simulink model "dlbsTestHarnessMatrixMultiply"  (R2025b)
settings: Solver=VariableStepAuto  StartTime=0.0  StopTime=10.0  RelTol=1e-3
undefined symbols (not defined in the file or in its folder): dY, W, X
libraries: dlbsBlockExtractGradientGF x2, dlbsBlockInsertGradientGF x1, dlbsBlockMatrixMultiply x1
settings Model: Creator=lt6037  LastModifiedBy=lt6037

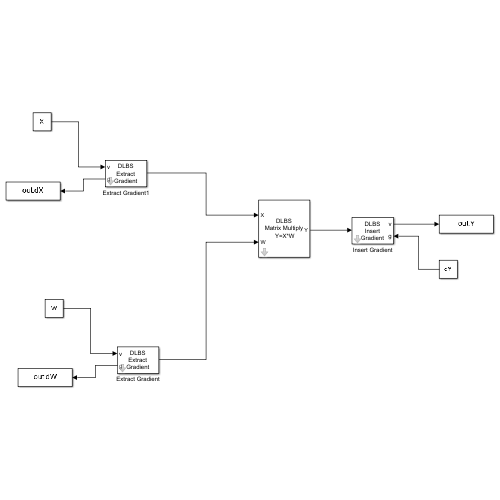
[thumbnail: Simulink's stored preview of the top-level diagram]
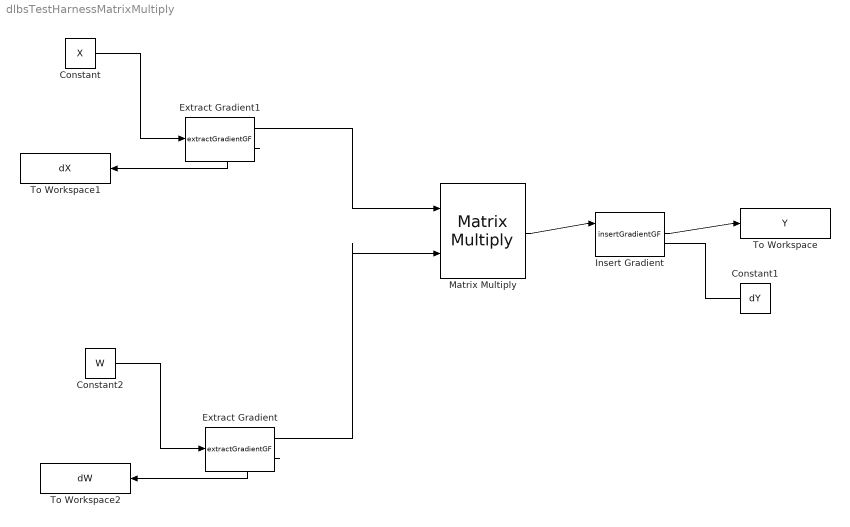
== system dlbsTestHarnessMatrixMultiply ==
  Constant : Constant  Value=X  VectorParams1D=off
  Constant1 : Constant  Value=dY  VectorParams1D=off
  Constant2 : Constant  Value=W  VectorParams1D=off
  Extract Gradient : dlbsBlockExtractGradientGF/extractGradientGF
  Extract Gradient1 : dlbsBlockExtractGradientGF/extractGradientGF
  Insert Gradient : dlbsBlockInsertGradientGF/insertGradientGF
  Matrix Multiply : dlbsBlockMatrixMultiply/Matrix Multiply
  To Workspace : ToWorkspace  VariableName=Y  SaveFormat=Timeseries  SampleTime=-1
      settings: MaxDataPoints=1
  To Workspace1 : ToWorkspace  VariableName=dX  SaveFormat=Timeseries  SampleTime=-1
      settings: MaxDataPoints=1
  To Workspace2 : ToWorkspace  VariableName=dW  SaveFormat=Timeseries  SampleTime=-1
      settings: MaxDataPoints=1
  wires:
  Extract Gradient1/2 -> To Workspace1/1
  Constant1/1 -> Insert Gradient/2
  Constant/1 -> Extract Gradient1/1
  Insert Gradient/1 -> To Workspace/1
  Extract Gradient/2 -> To Workspace2/1
  Constant2/1 -> Extract Gradient/1
  Extract Gradient1/1 -> Matrix Multiply/1
  Extract Gradient/1 -> Matrix Multiply/2
  Matrix Multiply/1 -> Insert Gradient/1
